simulink subsystem "featureExtraction"  (R2021a)
settings: Solver=VariableStepAuto  StartTime=0.0  StopTime=10.0  RelTol=1e-3
libraries: hdlsllib x10
settings Model: Creator=trevvvy  LastModifiedBy=trevvvy

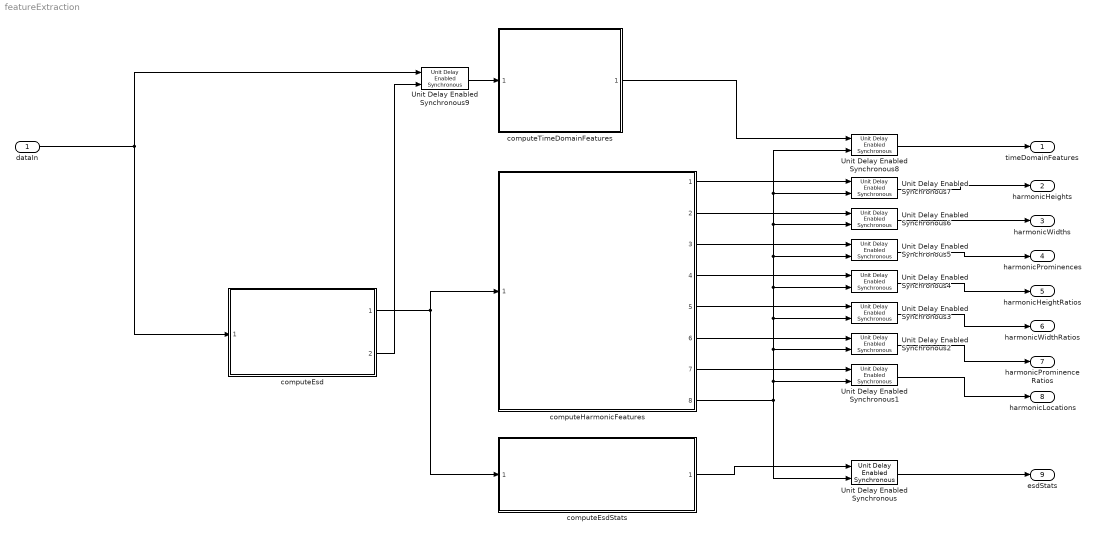
== system featureExtraction ==
  dataIn : Inport
  Unit Delay Enabled Synchronous{,1..9} (10 alike) : hdlsllib/Discrete/Unit Delay Enabled Synchronous  InitialCondition=0.0  SampleTime=-1
      settings: SourceProductBaseCode=SL
  computeEsd : Subsystem  ReferencedSubsystem=ESD
  computeEsdStats : Subsystem  ReferencedSubsystem=extractEsdStats
  computeHarmonicFeatures : Subsystem  ReferencedSubsystem=harmonicFeatures
  computeTimeDomainFeatures : Subsystem  ReferencedSubsystem=timeDomainFeatures
  timeDomainFeatures : Outport
  harmonicHeights : Outport  Port=2
  harmonicWidths : Outport  Port=3
  harmonicProminences : Outport  Port=4
  harmonicHeightRatios : Outport  Port=5
  harmonicWidthRatios : Outport  Port=6
  harmonicProminenceRatios : Outport  Port=7
  harmonicLocations : Outport  Port=8
  esdStats : Outport  Port=9
  wires:
  computeHarmonicFeatures/6 -> Unit Delay Enabled Synchronous2/1
  Unit Delay Enabled Synchronous3/1 -> harmonicWidthRatios/1
  Unit Delay Enabled Synchronous8/1 -> timeDomainFeatures/1
  computeEsd/1 -> computeHarmonicFeatures/1, computeEsdStats/1
  computeTimeDomainFeatures/1 -> Unit Delay Enabled Synchronous8/1
  computeHarmonicFeatures/7 -> Unit Delay Enabled Synchronous1/1
  computeHarmonicFeatures/5 -> Unit Delay Enabled Synchronous3/1
  dataIn/1 -> Unit Delay Enabled Synchronous9/1, computeEsd/1
  Unit Delay Enabled Synchronous7/1 -> harmonicHeights/1
  computeEsdStats/1 -> Unit Delay Enabled Synchronous/1
  Unit Delay Enabled Synchronous/1 -> esdStats/1
  Unit Delay Enabled Synchronous5/1 -> harmonicProminences/1
  Unit Delay Enabled Synchronous6/1 -> harmonicWidths/1
  Unit Delay Enabled Synchronous4/1 -> harmonicHeightRatios/1
  Unit Delay Enabled Synchronous2/1 -> harmonicProminenceRatios/1
  computeHarmonicFeatures/3 -> Unit Delay Enabled Synchronous5/1
  computeHarmonicFeatures/2 -> Unit Delay Enabled Synchronous6/1
  computeHarmonicFeatures/8 -> Unit Delay Enabled Synchronous1/2, Unit Delay Enabled Synchronous2/2, Unit Delay Enabled Synchronous3/2, Unit Delay Enabled Synchronous4/2, Unit Delay Enabled Synchronous5/2, Unit Delay Enabled Synchronous6/2, Unit Delay Enabled Synchronous7/2, Unit Delay Enabled Synchronous8/2, Unit Delay Enabled Synchronous/2
  computeHarmonicFeatures/4 -> Unit Delay Enabled Synchronous4/1
  computeEsd/2 -> Unit Delay Enabled Synchronous9/2
  Unit Delay Enabled Synchronous1/1 -> harmonicLocations/1
  Unit Delay Enabled Synchronous9/1 -> computeTimeDomainFeatures/1
  computeHarmonicFeatures/1 -> Unit Delay Enabled Synchronous7/1
